simulink model "platformODE"  (R2018b)
settings: Solver=VariableStepAuto  StartTime=0.0  StopTime=tsim  RelTol=1e-3
values from neighbouring files (symbols this model uses):
  initial_x0 = cat(1,initialR_s,initialR_m,initialV_s,initialV_m)    [Platform.m]
settings Model: Creator=Erin B  LastModifiedBy=embeato2

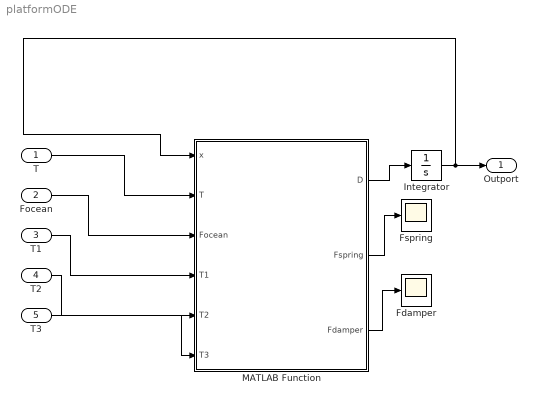
== system platformODE ==
  T : Inport  OutDataTypeStr=double  PortDimensions=3
  Focean : Inport  Port=2  PortDimensions=3
  T1 : Inport  Port=3  PortDimensions=3
  T2 : Inport  Port=4  PortDimensions=3
  T3 : Inport  Port=5  PortDimensions=3
  Fdamper : Scope
  Fspring : Scope
  Integrator : Integrator  InitialCondition=initial_x0
  MATLAB Function : MATLAB Function  TreatAsAtomicUnit=on
  Outport : Outport
  wires:
  MATLAB Function/1(D) -> Integrator/1
  Integrator/1 -> Outport/1, MATLAB Function/1(x)
  T/1 -> MATLAB Function/2(T)
  Focean/1 -> MATLAB Function/3(Focean)
  T1/1 -> MATLAB Function/4(T1)
  T2/1 -> MATLAB Function/5(T2)
  MATLAB Function/2(Fspring) -> Fspring/1
  MATLAB Function/3(Fdamper) -> Fdamper/1
  T3/1 -> MATLAB Function/6(T3)

== matlab function platformODE/MATLAB Function ==
  data: D output; x input; T input; Focean input; T1 input; T2 input; T3 input; system_param parameter; Fspring output; Fdamper output
function [D, Fspring, Fdamper] = sprungODE(x,T,Focean,T1,T2,T3, system_param)

D = NaN*x;
k = system_param.k;
b = system_param.b;
ms = system_param.ms;
g = system_param.g;
m = system_param.m;
rho = system_param.rho;
V = system_param.V;
h = system_param.h;
Vs = system_param.Vs;
lus = system_param.lus;

grav = [0;0;-g];
bouy = [0;0;rho*V*g];

R_s0 = x(1:3);
R_m0 = x(4:6);
V_s0 = x(7:9);
V_m0 = x(10:12);
R_sm = R_s0 - R_m0;
V_sm = V_s0 - V_m0;

D(1:3) = V_s0;
D(4:6) = V_m0;

Fspring = (k)*(norm(R_sm)-lus).*((R_sm)./norm(R_sm));
Fdamper = (b)*(norm(V_sm)).*((R_sm)./norm(R_sm));

D(7:9) = (1/ms).*(- Fspring - Fdamper + T + ms.*grav);
D(10:12) = (1/m).*(Focean + T1 + T2 + T3 + Fspring + Fdamper + m.*grav + bouy);


end
